simulink model "SegundaOrdemDominioDoTempoModel"  (R2019b)
settings: Solver=VariableStepAuto  StartTime=0.0  StopTime=tfinal  MaxStep=tStepMax  RelTol=1e-3
values from neighbouring files (symbols this model uses):
  beta = 2.*e.*w    [SegundaOrdemDominioDoTempoScript.m]
  Const = 0    [SegundaOrdemDominioDoTempoScript.m]
  omega = w.^2    [SegundaOrdemDominioDoTempoScript.m]
  omega1 = w1.^2    [SegundaOrdemDominioDoTempoScript.m]
  theta0 = 0    [SegundaOrdemDominioDoTempoScript.m]
  thetaDot0 = 0    [SegundaOrdemDominioDoTempoScript.m]
settings Model: Creator=pedro  LastModifiedBy=pedro

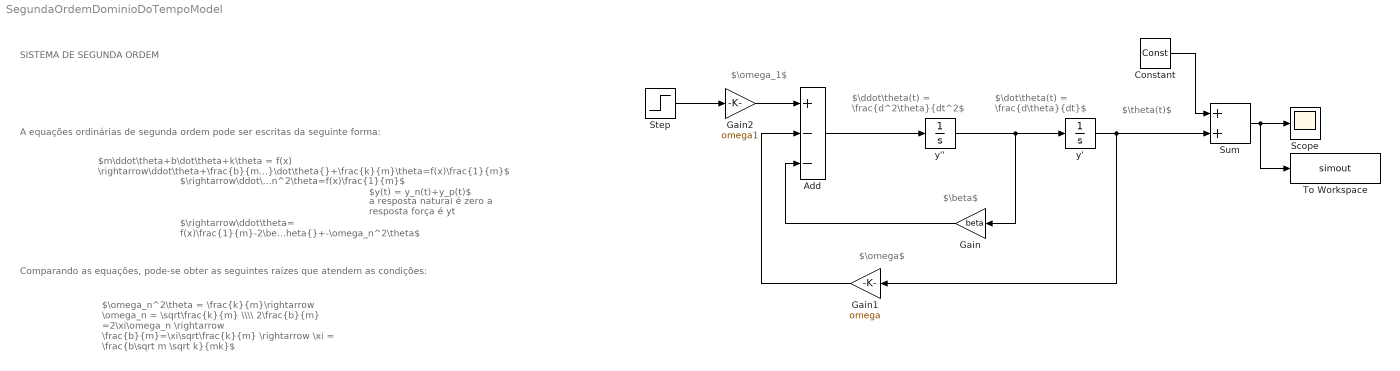
== system SegundaOrdemDominioDoTempoModel ==
  note: a resposta natural é zero
      | a resposta força é yt
  note: $\ddot\theta(t) = \frac{d^2\theta}{dt^2$
  note: SISTEMA DE SEGUNDA ORDEM
  note: $m\ddot\theta+b\dot\theta+k\theta = f(x) \rightarrow\ddot\theta+\frac{b}{m}\dot\theta{}+\frac{k}{m}\theta=f(x)\frac{1}{m}$
  note: Comparando as equações, pode-se obter as seguintes raízes que atendem as condições:
  note: A equações ordinárias de segunda ordem pode ser escritas da seguinte forma:
  note: $\omega_n^2\theta = \frac{k}{m}\rightarrow \omega_n = \sqrt\frac{k}{m} \\\\ 2\frac{b}{m} =2\xi\omega_n \rightarrow \frac{b}{m}=\xi\sqrt\frac{k}{m} \rightarrow \xi = \frac{b\sqrt m \sqrt k}{mk}$
  note: $\rightarrow\ddot\theta+2\beta\dot\theta{}+\omega_n^2\theta=f(x)\frac{1}{m}$
  note: $\dot\theta(t) = \frac{d\theta}{dt}$
  note: $\theta(t)$
  note: $\omega$
  note: $\beta$
  note: $\rightarrow\ddot\theta= f(x)\frac{1}{m}-2\beta\dot\theta{}+-\omega_n^2\theta$
  note: $y(t) = y_n(t)+y_p(t)$
  note: $\omega_1$
  Add : Sum  Inputs=+--
  Constant : Constant  Value=Const
  Gain : Gain  Gain=beta
  Gain1 : Gain  Gain=omega
  Gain2 : Gain  Gain=omega1
  Scope : Scope
  Step : Step  SampleTime=0
  Sum : Sum
  To Workspace : ToWorkspace  VariableName=simout  SampleTime=-1
      settings: Save2DSignal=2-D array (concatenate along first dimension)
  y' : Integrator  InitialCondition=theta0
  y'' : Integrator  InitialCondition=thetaDot0
  wires:
  Add/1 -> y''/1
  y''/1 -> Gain/1, y'/1
  y'/1 -> Sum/2, Gain1/1
  Gain/1 -> Add/3
  Gain1/1 -> Add/2
  Constant/1 -> Sum/1
  Step/1 -> Gain2/1
  Gain2/1 -> Add/1
  Sum/1 -> To Workspace/1, Scope/1
